simulink model "potentiometer"  (R2024b)
settings: Solver=FixedStepAuto  StartTime=0.0  StopTime=inf  RelTol=1e-3  EnableMultiTasking=on
libraries: stm32f4xxblockslib x2
settings Model: STM32="{\"AnalogInput\":[{\"ID\":\"untitled:1\"},{\"ID\":\"potentiometer:3\"}],\"DigitalPortRead\":{\"ID\":\"potentiometer:22\"}}"  Creator=spwkp  LastModifiedBy=spwkp
settings OptimizationCC: DefaultParameterBehavior=Inlined  EnhancedBackFolding=on  PassReuseOutputArgsAs=Individual arguments  ZeroExternalMemoryAtStartup=off  ZeroInternalMemoryAtStartup=off  MaxStackSize=512  OptimizeBlockOrder=speed  DifferentSizesBufferReuse=on  OptimizationCustomize=off  EfficientTunableParamExpr=on
settings DebuggingCC: ParameterTunabilityLossMsg=error
settings HardwareCC: ProdBitPerPointer=32  ProdBitPerSizeT=32  ProdBitPerPtrDiffT=32  ProdLargestAtomicInteger=Long  ProdLargestAtomicFloat=Double  ProdWordSize=32  ProdLongLongMode=on  ProdHWDeviceType=ARM Compatible->ARM Cortex-M
settings SFSimCC: MATLABDynamicMemAlloc=off
settings RTWCC: Description=Embedded Coder  SystemTargetFile=ert.tlc  HardwareBoard=STM32G4xx Based  TemplateMakefile=ert_default_tmf  Toolchain=GNU Tools for ARM Embedded Processors
settings CodeAppCC: ForceParamTrailComments=on  IgnoreCustomStorageClasses=off  OperatorAnnotations=on  SimulinkDataObjDesc=on  SFDataObjDesc=on  InsertBlockDesc=on
settings ERTTargetCC: TargetLangStandard=C99 (ISO)  CodeReplacementLibrary=ARM Cortex-M  ExtModeTransport=3  ExtModeStaticAlloc=on  ExtModeStaticAllocSize=2048  ExtModeMexFile=ext_xcp  ExtModeIntrfLevel=Level2 - Open

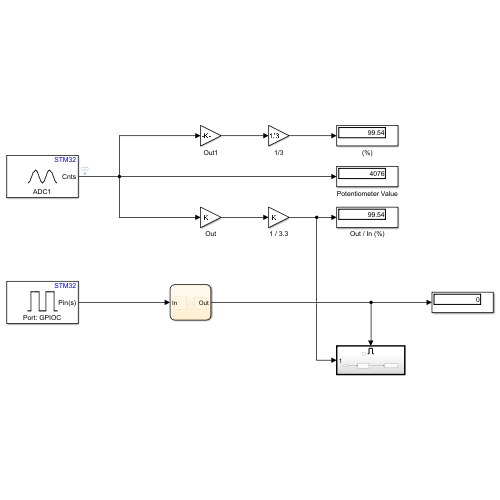
[thumbnail: Simulink's stored preview of the top-level diagram]
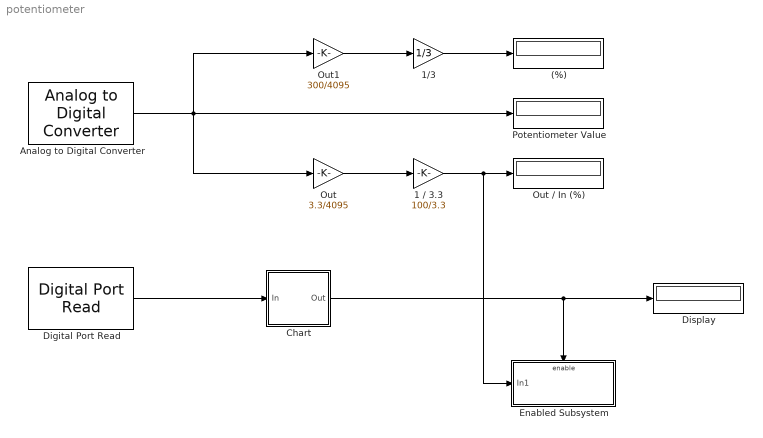
== system potentiometer ==
  (%) : Display
  1 / 3.3 : Gain  Gain=100/3.3
  1/3 : Gain  Gain=1/3
  Analog to Digital Converter : stm32f4xxblockslib/Analog to Digital Converter  ADCModule=ADC1  ConversionGroup=Regular  TriggerMode=Trigger and read  NumberOfConversions=1  EnableBufferConv=off  BufferLength=1  OutputStatus=off  SampleTime=-1  EnableSimPort=off  hoistedMaskSrc=ECSoC/ECSimCodegen/Analog to Digital Converter
  Chart : Stateflow chart  TreatAsAtomicUnit=on
  Digital Port Read : stm32f4xxblockslib/Digital Port Read  PortName=GPIOC  PinNumber=13  ReadOperation=on  IOAsArray=on  SampleTime=-1  EnableSimPort=off  hoistedMaskSrc=ECSoC/ECSimCodegen/Digital Port Read
      settings: LibrarySourceBlock=stm32g4xxblockslib/Digital Port Read
  Display : Display
  Enabled Subsystem : Subsystem  TreatAsAtomicUnit=on
  Out : Gain  Gain=3.3/4095
  Out / In (%) : Display
  Out1 : Gain  Gain=300/4095
  Potentiometer Value : Display
  wires:
  Out/1 -> 1 / 3.3/1
  Analog to Digital Converter/1 -> Out1/1, Out/1, Potentiometer Value/1
  1/3/1 -> (%)/1
  Out1/1 -> 1/3/1
  1 / 3.3/1 -> Enabled Subsystem/1(In1), Out / In (%)/1
  Digital Port Read/1 -> Chart/1(In)
  Chart/1(Out) -> Display/1, Enabled Subsystem/Enable

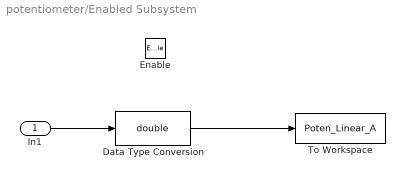
== system potentiometer/Enabled Subsystem ==
  In1 : Inport
  Enable : EnablePort
  Data Type Conversion : DataTypeConversion  OutDataTypeStr=double  SaturateOnIntegerOverflow=off  RndMeth=Floor
  To Workspace : ToWorkspace  VariableName=Poten_Linear_A  SampleTime=-1
      settings: Save2DSignal=2-D array (concatenate along first dimension)
  wires:
  In1/1 -> Data Type Conversion/1
  Data Type Conversion/1 -> To Workspace/1

== stateflow chart potentiometer/Chart ==
  state init
    In;
    Out = 0;
    Count = 1;
  state Log_dtat
    entry:
    during:
    Count = Count + 1;
    Out = 1;
    exit:
    Out = 0;
  (default) -> init
  Log_dtat -> init : [Count > 1000]
  init -> Log_dtat : [In == 1]
  data: In input; Out output; Count local
